simulink model "quaternion_simulation"  (R2022a)
settings: Solver=FixedStepAuto  StartTime=0.0  StopTime=60  FixedStep=Ts  RelTol=1e-3
values from neighbouring files (symbols this model uses):
  J_uav = diag([0.0118976 0.0118976 0.0218816])    [quaternion_simulation_init.m]
  K_att = [diag([100 100 3.16e-6]) diag([14.142 14.142 2.51e-3])]    [quaternion_simulation_init.m]
  K_pos = [diag([3.1622 3.1622 3.1622]) diag([2.7063 2.7063 2.7603])]    [quaternion_simulation_init.m]
  m_uav = 1.3    [quaternion_simulation_init.m]
  Ts = 0.005    [quaternion_simulation_init.m]
undefined symbols (not defined in the file or in its folder): sigbuilder_block
libraries: sharedtransform x2, SignalEditorBlockLib x1, uavutilslib x1
settings Model: PacingRate=3  Creator=marti  LastModifiedBy=martin
settings SolverCC: AlgebraicLoopSolver=TrustRegion
settings DebuggingCC: UnconnectedInputMsg=warning  UnconnectedOutputMsg=warning  UnconnectedLineMsg=warning  SFMachineParentedDataDiag=warning
settings RTWCC: DLArmComputeVersion=19.05

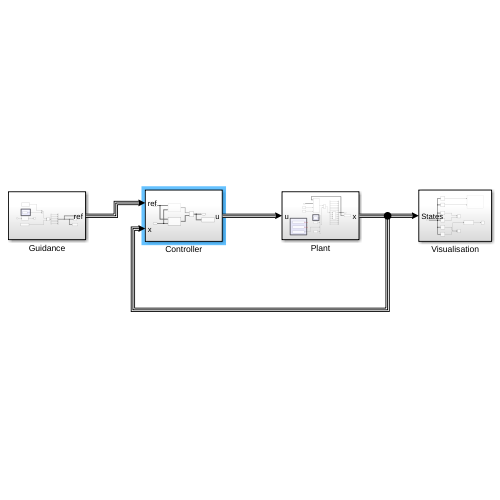
[thumbnail: Simulink's stored preview of the top-level diagram]
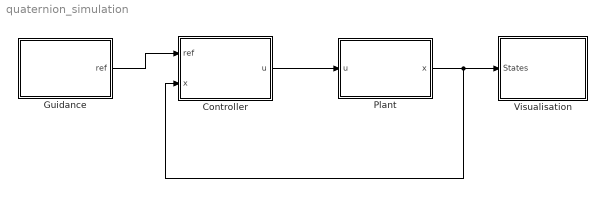
== system quaternion_simulation ==
  Controller : Subsystem
  Guidance : Subsystem
  Plant : Subsystem
  Visualisation : Subsystem
  wires:
  Guidance/1(ref) -> Controller/1(ref)
  Plant/1(x) -> Controller/2(x), Visualisation/1(States)
  Controller/1(u) -> Plant/1(u)

== system quaternion_simulation/Controller ==
  ref : Inport
  x : Inport  Port=2
  ADRC : Subsystem
  Manual Switch : ManualSwitch
  State-Feedback : Subsystem
  To Workspace : ToWorkspace  VariableName=control  SaveFormat=Timeseries  SampleTime=-1
  u : Outport
  wires:
  x/1 -> ADRC/2(x), State-Feedback/2(x)
  ref/1 -> State-Feedback/1(ref), ADRC/1(ref)
  ADRC/1(u) -> Manual Switch/2
  State-Feedback/1(u) -> Manual Switch/1
  Manual Switch/1 -> u/1, To Workspace/1

== system quaternion_simulation/Guidance ==
  note: velocity setpoints
  Bus Creator : BusCreator  Inputs=6
  Clock : Clock
  Constant : Constant  Value=[0;0;0]
  Demux : Demux  Outputs=6
  Fixed Setpoint : Constant  Value=[0; 0; 0; 0; 0; 0]
  Manual Switch : ManualSwitch  CurrentSetting=0
  Mux : Mux  Inputs=2
  Signal Editor : SignalEditorBlockLib/Signal Editor  FileName=/home/martin/thesis/ADRC_examples/Quaternion Simulation/trajectory.mat  ActiveScenario=square_1m_trajectory  ActiveSignal=Setpoint  IsBus=off  OutputBusObjectStr=Bus: BusObject  SampleTime=0  Interpolate=off  ZeroCross=off  OutputAfterFinalValue=Setting to zero  Unit=inherit  PreserveSignalName=on
  Terminator : Terminator
  To Workspace : ToWorkspace  VariableName=setpoints  SaveFormat=Timeseries  SampleTime=-1
  Trajectory : Scope
  Trajectory Generator : MATLAB Function  TreatAsAtomicUnit=on
  Out Bus Element : Outport  PortName=ref
  wires:
  Fixed Setpoint/1 -> Manual Switch/2
  Clock/1 -> Trajectory Generator/1(t)
  Constant/1 -> Mux/2
  Signal Editor/1 -> Mux/1
  Mux/1 -> Manual Switch/1
  Trajectory Generator/1(x_d) -> Terminator/1
  Manual Switch/1 -> Demux/1
  Demux/1 -> Bus Creator/1  "X"
  Demux/2 -> Bus Creator/2  "Y"
  Demux/3 -> Bus Creator/3  "Z"
  Demux/4 -> Bus Creator/4  "dX"
  Demux/5 -> Bus Creator/5  "dY"
  Demux/6 -> Bus Creator/6  "dZ"
  Bus Creator/1 -> Out Bus Element/1, To Workspace/1, Trajectory/1

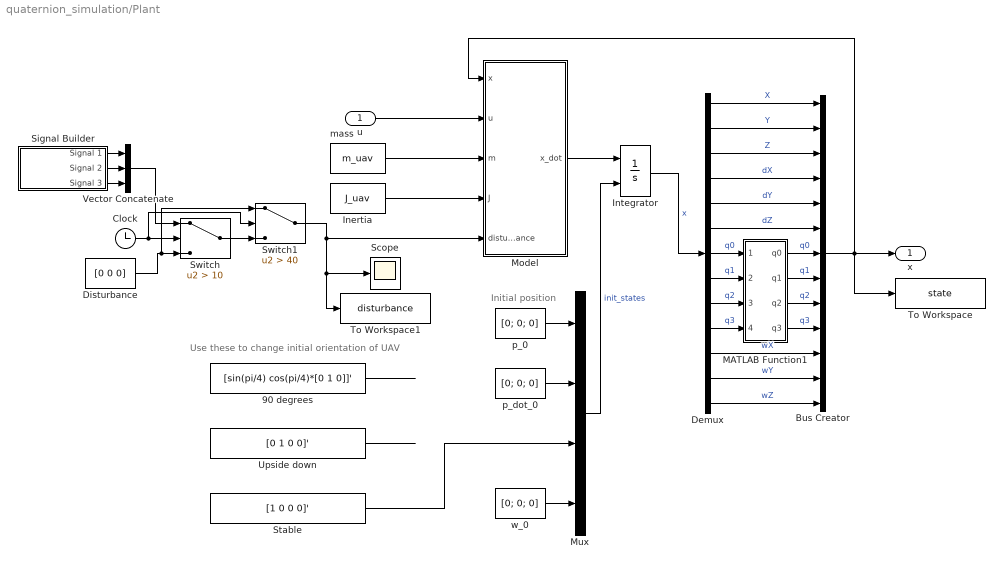
== system quaternion_simulation/Plant ==
  note: Initial position
  note: Use these to change initial orientation of UAV
  u : Inport
  90 degrees : Constant  Value=[sin(pi/4) cos(pi/4)*[0 1 0]]'  VectorParams1D=off
  Bus Creator : BusCreator  Inputs=13
  Clock : Clock
  Demux : Demux  Outputs=13
  Disturbance : Constant  Value=[0 0 0]  VectorParams1D=off
  Inertia : Constant  Value=J_uav  VectorParams1D=off
  Integrator : Integrator  InitialConditionSource=external
  MATLAB Function1 : MATLAB Function  TreatAsAtomicUnit=on
  Model : MATLAB Function  TreatAsAtomicUnit=on
  Mux : Mux
  Scope : Scope
  Signal Builder : Subsystem  Tag=STV Subsys  LoadFcn=sigbuilder_block('load');  StartFcn=sigbuilder_block('start');  StopFcn=sigbuilder_block('stop');  ClipboardFcn=sigbuilder_block('clipboard');  mask(Sigbuilder block){tuvar=[0:10]}
      mask help: Simulink:masks:SigbuilderBlock_MD
      mask init:
      | if ~strcmp(get_param(bdroot(gcbh),'SimulationStatus'),'stopped') tuvar = sigbuilder_block('maskInit'); end
      settings: CopyFcn=sigbuilder_block('copy');  DeleteFcn=sigbuilder_block('delete');  ModelCloseFcn=sigbuilder_block('modelClose');  PreSaveFcn=sigbuilder_block('preSave');  PauseFcn=sigbuilder_block('pause');  ContinueFcn=sigbuilder_block('continue');  NameChangeFcn=sigbuilder_block('namechange');  OpenFcn=sigbuilder_block('open',[437.6 3 550.4 399.75 ]);  CloseFcn=sigbuilder_block('close');
      mask Display: plot(0, 0, 100, 100,[2, 2, 32, 32, 2], [68, 8, 8, 68, 68],[32, 2], [38, 38], [32, 19, 2],[53, 60, 44], [32, 17, 17, 2],[16, 16, 31, 31]);txt = getActiveGroup(gcbh);text(2, 100, txt,'verticalAlignment', 'top');
  Stable : Constant  Value=[1 0 0 0]'  VectorParams1D=off
  Switch : Switch  Criteria=u2 > Threshold  Threshold=10  SaturateOnIntegerOverflow=off  InputSameDT=off
  Switch1 : Switch  Criteria=u2 > Threshold  Threshold=40  SaturateOnIntegerOverflow=off  InputSameDT=off
  To Workspace : ToWorkspace  VariableName=state  SaveFormat=Timeseries  SampleTime=-1
  To Workspace1 : ToWorkspace  VariableName=disturbance  SaveFormat=Timeseries  SampleTime=-1
  Upside down : Constant  Value=[0 1 0 0]'  VectorParams1D=off
  Vector Concatenate : Concatenate  NumInputs=3  Mode=Multidimensional array  ConcatenateDimension=2
  mass : Constant  Value=m_uav
  p_0 : Constant  Value=[0; 0; 0]  VectorParams1D=off
  p_dot_0 : Constant  Value=[0; 0; 0]  VectorParams1D=off
  w_0 : Constant  Value=[0; 0; 0]  VectorParams1D=off
  x : Outport
  wires:
  Inertia/1 -> Model/4(J)
  Model/1(x_dot) -> Integrator/1
  p_0/1 -> Mux/1
  p_dot_0/1 -> Mux/2
  w_0/1 -> Mux/4
  Integrator/1 -> Demux/1  "x"
  u/1 -> Model/2(u)
  Mux/1 -> Integrator/2  "init_states"
  Bus Creator/1 -> Model/1(x), To Workspace/1, x/1
  Demux/1 -> Bus Creator/1  "X"
  Demux/13 -> Bus Creator/13  "wZ"
  Demux/2 -> Bus Creator/2  "Y"
  Demux/3 -> Bus Creator/3  "Z"
  Demux/4 -> Bus Creator/4  "dX"
  Demux/5 -> Bus Creator/5  "dY"
  Demux/6 -> Bus Creator/6  "dZ"
  Demux/11 -> Bus Creator/11  "wX"
  Demux/12 -> Bus Creator/12  "wY"
  Demux/7 -> MATLAB Function1/1(q0_in)  "q0"
  Demux/8 -> MATLAB Function1/2(q1_in)  "q1"
  Demux/9 -> MATLAB Function1/3(q2_in)  "q2"
  Demux/10 -> MATLAB Function1/4(q3_in)  "q3"
  MATLAB Function1/1(q0) -> Bus Creator/7  "q0"
  MATLAB Function1/2(q1) -> Bus Creator/8  "q1"
  MATLAB Function1/3(q2) -> Bus Creator/9  "q2"
  MATLAB Function1/4(q3) -> Bus Creator/10  "q3"
  Stable/1 -> Mux/3
  mass/1 -> Model/3(m)
  90 degrees/1 -> ?
  Upside down/1 -> ?
  Vector Concatenate/1 -> Switch/1
  Clock/1 -> Switch1/2, Switch/2
  Disturbance/1 -> Switch1/1, Switch/3
  Signal Builder/1(Signal 1) -> Vector Concatenate/1
  Signal Builder/2(Signal 2) -> Vector Concatenate/2
  Signal Builder/3(Signal 3) -> Vector Concatenate/3
  Switch/1 -> Switch1/3
  Switch1/1 -> To Workspace1/1, Scope/1, Model/5(disturbance)

== system quaternion_simulation/Visualisation ==
  States : Inport
  Euler : Scope
  Linear : Scope  NumInputPorts=2
  Quaternion : Scope  NumInputPorts=2
  Quaternions to Rotation Angles : sharedtransform/Quaternions to Rotation Angles  rotationOrder=XYZ  aMode=aMode
      settings: SourceProductBaseCode=AE,PW,DR,MT,VE
  Selector : Selector  InputPortWidth=13  IndexOptions=Index vector (dialog)  Indices=[1:3]  OutputSizes=1
  Selector1 : Selector  InputPortWidth=13  IndexOptions=Index vector (dialog)  Indices=[4:6]  OutputSizes=1
  Selector2 : Selector  InputPortWidth=13  IndexOptions=Index vector (dialog)  Indices=[7:10]  OutputSizes=1
  Selector3 : Selector  InputPortWidth=13  IndexOptions=Index vector (dialog)  Indices=[11:13]  OutputSizes=1
  Selector4 : Selector  InputPortWidth=13  IndexOptions=Index vector (dialog)  Indices=[1:3]  OutputSizes=1
  Selector5 : Selector  InputPortWidth=13  IndexOptions=Index vector (dialog)  Indices=[7:10]  OutputSizes=1
  UAV Animation : uavutilslib/UAV Animation  Commented=on  UAVType=Multirotor  UAVSize=1  InertialZDirection=Up  SampleTime=-1
      settings: SourceProductBaseCode=UV
  wires:
  Selector2/1 -> Quaternions to Rotation Angles/1, Quaternion/1  "Orientation"
  States/1 -> Selector4/1, Selector5/1, Selector/1, Selector3/1, Selector2/1, Selector1/1
  Selector1/1 -> Linear/2  "Velocity"
  Selector/1 -> Linear/1  "Position"
  Selector3/1 -> Quaternion/2  "Angular Velocity"
  Selector5/1 -> UAV Animation/2  "Rotation"
  Selector4/1 -> UAV Animation/1  "Translation"
  Quaternions to Rotation Angles/1 -> Euler/1

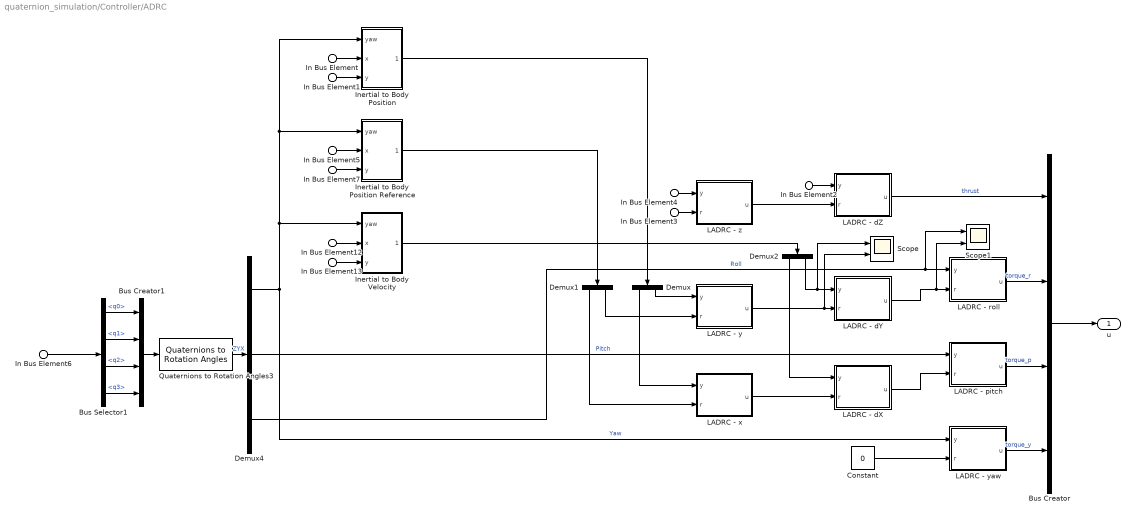
== system quaternion_simulation/Controller/ADRC ==
  In Bus Element7 : Inport  PortName=ref  Element=Y
  In Bus Element5 : Inport  PortName=ref  Element=X
  In Bus Element3 : Inport  PortName=ref  Element=Z
  In Bus Element6 : Inport  Port=2  PortName=x
  In Bus Element : Inport  Port=2  PortName=x  Element=X
  In Bus Element1 : Inport  Port=2  PortName=x  Element=Y
  In Bus Element12 : Inport  Port=2  PortName=x  Element=dX
  In Bus Element13 : Inport  Port=2  PortName=x  Element=dY
  In Bus Element4 : Inport  Port=2  PortName=x  Element=Z
  In Bus Element2 : Inport  Port=2  PortName=x  Element=dZ
  Bus Creator : BusCreator  Inputs=4
  Bus Creator1 : BusCreator  Inputs=4
  Bus Selector1 : BusSelector  OutputSignals=q0,q1,q2,q3
  Constant : Constant  Value=0
  Demux : Demux  Outputs=2
  Demux1 : Demux  Outputs=2
  Demux2 : Demux  Outputs=2
  Demux4 : Demux  Outputs=3
  Inertial to Body Position : Subsystem
  Inertial to Body Position Reference : Subsystem
  Inertial to Body Velocity : Subsystem
  LADRC - dX : Subsystem  VariantControl=Choice
  LADRC - dY : Subsystem  VariantControl=Choice
  LADRC - dZ : Subsystem  VariantControl=Choice
  LADRC - pitch : Subsystem  VariantControl=Choice
  LADRC - roll : Subsystem  VariantControl=Choice
  LADRC - x : Subsystem  VariantControl=Choice
  LADRC - y : Subsystem  VariantControl=Choice
  LADRC - yaw : Subsystem  VariantControl=Choice
  LADRC - z : Subsystem  VariantControl=Choice
  Quaternions to Rotation Angles3 : sharedtransform/Quaternions to Rotation Angles  rotationOrder=ZYX  aMode=aMode
      settings: SourceProductBaseCode=AE,PW,DR,MT,VE
  Scope : Scope  NumInputPorts=2
  Scope1 : Scope  NumInputPorts=2
  u : Outport
  wires:
  Bus Creator/1 -> u/1
  Demux4/3 -> Scope1/1, LADRC - roll/1(y)  "Roll"
  Bus Selector1/4 -> Bus Creator1/4  "<q3>"
  Bus Selector1/2 -> Bus Creator1/2  "<q1>"
  Bus Creator1/1 -> Quaternions to Rotation Angles3/1
  Bus Selector1/3 -> Bus Creator1/3  "<q2>"
  Bus Selector1/1 -> Bus Creator1/1  "<q0>"
  Demux4/1 -> LADRC - yaw/1(y), Inertial to Body Velocity/1(yaw), Inertial to Body Position/1(yaw), Inertial to Body Position Reference/1(yaw)  "Yaw"
  LADRC - dZ/1(u) -> Bus Creator/1  "thrust"
  Constant/1 -> LADRC - yaw/2(r)
  In Bus Element/1 -> Inertial to Body Position/2(x)
  In Bus Element1/1 -> Inertial to Body Position/3(y)
  In Bus Element13/1 -> Inertial to Body Velocity/3(y)
  LADRC - dY/1(u) -> Scope1/2, LADRC - roll/2(r)
  LADRC - dX/1(u) -> LADRC - pitch/2(r)
  In Bus Element6/1 -> Bus Selector1/1
  Quaternions to Rotation Angles3/1 -> Demux4/1  "ZYX"
  Demux4/2 -> LADRC - pitch/1(y)  "Pitch"
  Demux2/1 -> LADRC - dX/1(y)
  LADRC - yaw/1(u) -> Bus Creator/4  "torque_y"
  LADRC - pitch/1(u) -> Bus Creator/3  "torque_p"
  LADRC - roll/1(u) -> Bus Creator/2  "torque_r"
  In Bus Element3/1 -> LADRC - z/2(r)
  In Bus Element4/1 -> LADRC - z/1(y)
  In Bus Element5/1 -> Inertial to Body Position Reference/2(x)
  In Bus Element7/1 -> Inertial to Body Position Reference/3(y)
  In Bus Element12/1 -> Inertial to Body Velocity/2(x)
  LADRC - x/1(u) -> LADRC - dX/2(r)
  Inertial to Body Position/1(xy_body) -> Demux/1
  Demux/1 -> LADRC - x/1(y)
  Inertial to Body Position Reference/1(xy_body) -> Demux1/1
  Demux1/1 -> LADRC - x/2(r)
  Inertial to Body Velocity/1(xy_body) -> Demux2/1
  Demux2/2 -> Scope/1, LADRC - dY/1(y)
  LADRC - z/1(u) -> LADRC - dZ/2(r)
  LADRC - y/1(u) -> Scope/2, LADRC - dY/2(r)
  Demux1/2 -> LADRC - y/2(r)
  In Bus Element2/1 -> LADRC - dZ/1(y)
  Demux/2 -> LADRC - y/1(y)

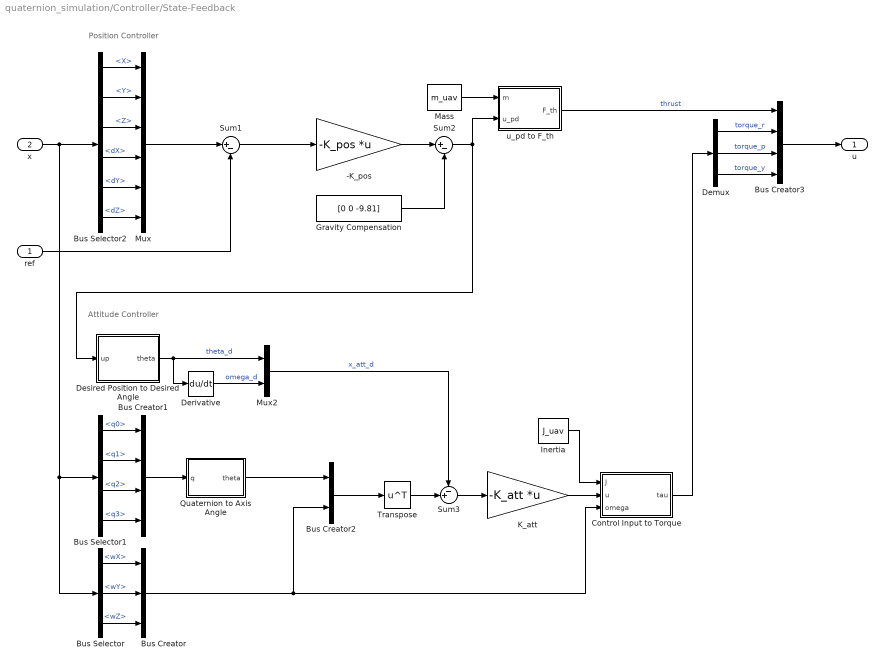
== system quaternion_simulation/Controller/State-Feedback ==
  note: Attitude Controller
  note: Position Controller
  ref : Inport
  x : Inport  Port=2
  -K_pos : Gain  Gain=-K_pos  Multiplication=Matrix(K*u) (u vector)
  Bus Creator : BusCreator  Inputs=3
  Bus Creator1 : BusCreator  Inputs=4
  Bus Creator2 : BusCreator  Inputs=2
  Bus Creator3 : BusCreator  Inputs=4
  Bus Selector : BusSelector  OutputSignals=wX,wY,wZ
  Bus Selector1 : BusSelector  OutputSignals=q0,q1,q2,q3
  Bus Selector2 : BusSelector  OutputSignals=X,Y,Z,dX,dY,dZ
  Control Input to Torque : MATLAB Function  TreatAsAtomicUnit=on
  Demux : Demux  Outputs=3
  Derivative : Derivative
  Desired Position to Desired Angle : MATLAB Function  TreatAsAtomicUnit=on
  Gravity Compensation : Constant  Value=[0 0 -9.81]
  Inertia : Constant  Value=J_uav  VectorParams1D=off
  K_att : Gain  Gain=-K_att  Multiplication=Matrix(K*u) (u vector)
  Mass : Constant  Value=m_uav
  Mux : Mux  Inputs=6
  Mux2 : Mux  Inputs=2
  Quaternion to Axis Angle : MATLAB Function  TreatAsAtomicUnit=on
  Sum1 : Sum  Inputs=|+-
  Sum2 : Sum  Inputs=|+-
  Sum3 : Sum  Inputs=-+|
  Transpose : Math  Operator=transpose
  u_pd to F_th : MATLAB Function  TreatAsAtomicUnit=on
  u : Outport
  wires:
  u_pd to F_th/1(F_th) -> Bus Creator3/1  "thrust"
  Bus Selector1/1 -> Bus Creator1/1  "<q0>"
  x/1 -> Bus Selector/1, Bus Selector1/1, Bus Selector2/1
  Bus Selector1/3 -> Bus Creator1/3  "<q2>"
  Bus Selector2/3 -> Mux/3  "<Z>"
  Bus Selector/3 -> Bus Creator/3  "<wZ>"
  Bus Selector2/1 -> Mux/1  "<X>"
  Bus Creator/1 -> Bus Creator2/2, Control Input to Torque/3(omega)
  Bus Selector2/6 -> Mux/6  "<dZ>"
  Bus Selector2/5 -> Mux/5  "<dY>"
  Bus Selector2/4 -> Mux/4  "<dX>"
  Bus Selector1/4 -> Bus Creator1/4  "<q3>"
  Bus Selector2/2 -> Mux/2  "<Y>"
  Bus Creator2/1 -> Transpose/1
  Bus Selector1/2 -> Bus Creator1/2  "<q1>"
  Quaternion to Axis Angle/1(theta) -> Bus Creator2/1
  Bus Selector/2 -> Bus Creator/2  "<wY>"
  Bus Selector/1 -> Bus Creator/1  "<wX>"
  Mass/1 -> u_pd to F_th/1(m)
  ref/1 -> Sum1/2
  Gravity Compensation/1 -> Sum2/2
  Sum2/1 -> u_pd to F_th/2(u_pd), Desired Position to Desired Angle/1(up)
  Sum1/1 -> -K_pos/1
  Mux/1 -> Sum1/1
  Inertia/1 -> Control Input to Torque/1(J)
  Bus Creator1/1 -> Quaternion to Axis Angle/1(q)
  -K_pos/1 -> Sum2/1
  Sum3/1 -> K_att/1
  K_att/1 -> Control Input to Torque/2(u)
  Control Input to Torque/1(tau) -> Demux/1
  Derivative/1 -> Mux2/2  "omega_d"
  Desired Position to Desired Angle/1(theta) -> Derivative/1, Mux2/1  "theta_d"
  Transpose/1 -> Sum3/2
  Mux2/1 -> Sum3/1  "x_att_d"
  Bus Creator3/1 -> u/1
  Demux/2 -> Bus Creator3/3  "torque_p"
  Demux/1 -> Bus Creator3/2  "torque_r"
  Demux/3 -> Bus Creator3/4  "torque_y"

== system quaternion_simulation/Plant/Signal Builder ==
  Demux : Demux  Tag=STV Demux  Outputs=3
      settings: DisplayOption=none
  FromWs : FromWorkspace  Tag=STV FromWs  VariableName=tuvar
      SigBuilderData=|
      | common.afterFinalStr = 'Extrapolate'
      | common.sampleTime = 0
      | dataSet.timeRange = [0 100]
      | dataSet.name = 'Group 1'
      | sbobj.Groups.Name = 'Group 1'
      | sbobj.Groups.Signals(1).Name = 'Signal 1'
      | sbobj.Groups.Signals(1).XData = [0 2 4 6 8 10 12 14 16 18 20 22 24 26 28 30 32 34 36 38 40 42 44 46 48 50 52 54 56 58 60 62 64 66 68 70 72 74 76 78 80 82 84 86 88 90 92 94 96 98 100]
      | sbobj.Groups.Signals(1).YData = [0.949221831131 0.307061919147 0.135174942099 0.515246335525 0.261406324055 -0.941485770955 -0.162337672804 -0.146054634332 -0.532011376809 1.68210359466 -0.87572934616 -0.48381505011 -0.712004549027 -1.17421233146 -0.192239517539 -0.274070229933 1.53007251442 -0.249024742514 -1.06421341289 1.60345729812 1.23467914689 -0.229626450963 -1.50615970398 -0.444627816447 -0.155941035725 0.276068253932 -0.261163645776 0.443421912904 0.391894209432 -1.25067890683 -0.947960922331 -0.74110609394 -0.507817550278 -0.3205755066 0.0124690413616 -3.0291773414 -0.457014640872 1.24244840639 -1.06670139898 0.933728162671 0.350321001356 -0.0290057637087 0.182452167506 -1.56505601415 -0.0845394798177 1.6039463506 0.0983477746401 0.0413736134896 -0.734169112697 -0.0308137300123 0.232347012624]
      | sbobj.Groups.Signals(2).Name = 'Signal 2'
      | sbobj.Groups.Signals(2).XData = [0 1 2 3 4 5 6 7 8 9 10 11 12 13 14 15 16 17 18 19 20 21 22 23 24 25 26 27 28 29 30 31 32 33 34 35 36 37 38 39 40 41 42 43 44 45 46 47 48 49 50 51 52 53 54 55 56 57 58 59 60 61 62 63 64 65 66 67 68 69 70 71 72 73 74 75 76 77 78 79 80 81 82 83 84 85 86 87 88 89 90 91 92 93 94 95 96 97 98 99 100]
      | sbobj.Groups.Signals(2).YData = [-0.888032082329 0.100092833139 -0.544528929991 0.303520794649 -0.600326562134 0.489965321174 0.739363123604 1.71188778298 -0.194123535758 -2.13835526944 -0.839588747337 1.354594328 -1.07215528838 0.960953869741 0.124049800003 1.43669662272 -1.96089999937 -0.197698225974 -1.20784548526 2.90800803073 0.825218894228 1.37897197792 -1.05818025799 -0.468615581101 -0.27246940925 1.09842461789 -0.277871932788 0.701541458163 -2.05181629991 -0.353849997774 -0.823586525157 -1.5770570228 0.507974650906 0.281984063671 0.0334798822445 -1.33367794343 1.12749227834 0.350179410603 -0.299066030333 0.0228897927516 -0.261995434966 -1.75021236845 -0.285650971595 -0.831366511568 -0.979206305167 -1.15640165566 -0.533557109316 -2.00263573588 0.964229422632 0.520060101455 -0.0200278516425 -0.0347710860285 -0.798163584564 1.01868528213 -0.133217479508 -0.714530163787 1.35138576843 -0.224771056053 -0.589029030721 -0.293753597735 -0.847926243638 -1.12012830124 2.52599969212 1.65549759289 0.307535159238 -1.25711835935 -0.865468030555 -0.176534114231 0.791416061629 -1.33200442132 -2.32986715581 -1.44909729284 0.333510833066 0.391353604433 0.451679418928 -0.130284653146 0.183689095862 -0.476153016619 0.862021611557 -1.36169447087 0.455029556444 -0.848709379934 -0.334886938964 0.552783345945 1.0390906535 -1.11763868327 1.26065870912 0.660143141047 -0.0678655535427 -0.195221197899 -0.217606350143 -0.303107621352 0.0230456244251 0.0512903558488 0.826062790212 1.52697668673 0.466914435685 -0.209713338389 0.625190357088 0.183227263001 -1.02976754357]
      | sbobj.Groups.Signals(3).Name = 'Signal 3'
      | sbobj.Groups.Signals(3).XData = [0 1 2 3 4 5 6 7 8 9 10 11 12 13 14 15 16 17 18 19 20 21 22 23 24 25 26 27 28 29 30 31 32 33 34 35 36 37 38 39 40 41 42 43 44 45 46 47 48 49 50 51 52 53 54 55 56 57 58 59 60 61 62 63 64 65 66 67 68 69 70 71 72 73 74 75 76 77 78 79 80 81 82 83 84 85 86 87 88 89 90 91 92 93 94 95 96 97 98 99 100]
      | sbobj.Groups.Signals(3).YData = [0.537667139546 1.8338850146 -2.258846861 0.862173320368 0.318765239859 -1.30768829631 -0.433592022306 0.342624466539 3.57839693973 2.76943702988 -1.34988694016 3.03492346633 0.725404224946 -0.0630548731897 0.714742903826 -0.2049660583 -0.124144348216 1.48969760779 1.4090344898 1.41719241343 0.671497133608 -1.20748692269 0.717238651329 1.63023528916 0.488893770312 1.03469300992 0.726885133383 -0.303440924786 0.293871467097 -0.787282803759 0.888395631758 -1.14707010697 -1.06887045817 -0.809498694425 -2.94428416199 1.43838029282 0.325190539456 -0.75492831917 1.3702985401 -1.71151641885 -0.102242446085 -0.241447041607 0.319206739166 0.312858596637 -0.864879917324 -0.0300512961963 -0.164879019209 0.627707287529 1.09326566904 1.10927329761 -0.863652821989 0.0773590911304 -1.21411704362 -1.11350074149 -0.00684932810335 1.53263030828 -0.769665913754 0.37137881276 -0.225584402271 1.11735613881 -1.08906429505 0.032557464165 0.552527021112 1.10061021788 1.5442118955 0.0859311331754 -1.49159031064 -0.74230183726 -1.06158173332 2.350457224 -0.615601881467 0.748076783704 -0.192418510588 0.888610425421 -0.764849236568 -1.40226896934 -1.42237592509 0.48819390986 -0.177375156619 -0.196053487807 1.41931015064 0.291584373984 0.197811053464 1.58769908997 -0.80446595635 0.69662441585 0.835088165073 -0.243715140378 0.215670086404 -1.16584393148 -1.1479527789 0.104874716016 0.722254032225 2.58549125262 -0.666890670701 0.187331024579 -0.082494425371 -1.93302291785 -0.438966153935 -1.79467884146 0.840375529754]
      | sbobj.Groups.TimeRange = [0 100]
  Signal 1 : Outport  Tag=STV Outport
  Signal 2 : Outport  Tag=STV Outport  Port=2
  Signal 3 : Outport  Tag=STV Outport  Port=3
  wires:
  Demux/1 -> Signal 1/1
  FromWs/1 -> Demux/1
  Demux/2 -> Signal 2/1
  Demux/3 -> Signal 3/1

== system quaternion_simulation/Controller/ADRC/Inertial to Body Position ==
  yaw : Inport
  x : Inport  Port=2
  y : Inport  Port=3
  Gain : Gain  Gain=-1
  Matrix Concatenate : Concatenate  Mode=Multidimensional array  ConcatenateDimension=2
  MatrixMultiply : Product  Multiplication=Matrix(*)
  Trigonometric Function : Trigonometry  Operator=sincos
  Vector Concatenate : Concatenate
  Vector Concatenate1 : Concatenate
  Vector Concatenate2 : Concatenate
  xy_body : Outport
  wires:
  Trigonometric Function/2 -> Vector Concatenate1/2, Vector Concatenate/1
  Trigonometric Function/1 -> Vector Concatenate1/1, Gain/1
  Gain/1 -> Vector Concatenate/2
  Matrix Concatenate/1 -> MatrixMultiply/1
  MatrixMultiply/1 -> xy_body/1
  Vector Concatenate2/1 -> MatrixMultiply/2
  Vector Concatenate/1 -> Matrix Concatenate/1
  Vector Concatenate1/1 -> Matrix Concatenate/2
  y/1 -> Vector Concatenate2/2
  x/1 -> Vector Concatenate2/1
  yaw/1 -> Trigonometric Function/1

== system quaternion_simulation/Controller/ADRC/Inertial to Body Position Reference ==
  yaw : Inport
  x : Inport  Port=2
  y : Inport  Port=3
  Gain : Gain  Gain=-1
  Matrix Concatenate : Concatenate  Mode=Multidimensional array  ConcatenateDimension=2
  MatrixMultiply : Product  Multiplication=Matrix(*)
  Trigonometric Function : Trigonometry  Operator=sincos
  Vector Concatenate : Concatenate
  Vector Concatenate1 : Concatenate
  Vector Concatenate2 : Concatenate
  xy_body : Outport
  wires:
  Trigonometric Function/2 -> Vector Concatenate1/2, Vector Concatenate/1
  Trigonometric Function/1 -> Vector Concatenate1/1, Gain/1
  Gain/1 -> Vector Concatenate/2
  Matrix Concatenate/1 -> MatrixMultiply/1
  MatrixMultiply/1 -> xy_body/1
  Vector Concatenate2/1 -> MatrixMultiply/2
  Vector Concatenate/1 -> Matrix Concatenate/1
  Vector Concatenate1/1 -> Matrix Concatenate/2
  y/1 -> Vector Concatenate2/2
  x/1 -> Vector Concatenate2/1
  yaw/1 -> Trigonometric Function/1

== system quaternion_simulation/Controller/ADRC/Inertial to Body Velocity ==
  yaw : Inport
  x : Inport  Port=2
  y : Inport  Port=3
  Gain : Gain  Gain=-1
  Matrix Concatenate : Concatenate  Mode=Multidimensional array  ConcatenateDimension=2
  MatrixMultiply : Product  Multiplication=Matrix(*)
  Trigonometric Function : Trigonometry  Operator=sincos
  Vector Concatenate : Concatenate
  Vector Concatenate1 : Concatenate
  Vector Concatenate2 : Concatenate
  xy_body : Outport
  wires:
  Trigonometric Function/2 -> Vector Concatenate1/2, Vector Concatenate/1
  Trigonometric Function/1 -> Vector Concatenate1/1, Gain/1
  Gain/1 -> Vector Concatenate/2
  Matrix Concatenate/1 -> MatrixMultiply/1
  MatrixMultiply/1 -> xy_body/1
  Vector Concatenate2/1 -> MatrixMultiply/2
  Vector Concatenate/1 -> Matrix Concatenate/1
  Vector Concatenate1/1 -> Matrix Concatenate/2
  y/1 -> Vector Concatenate2/2
  x/1 -> Vector Concatenate2/1
  yaw/1 -> Trigonometric Function/1

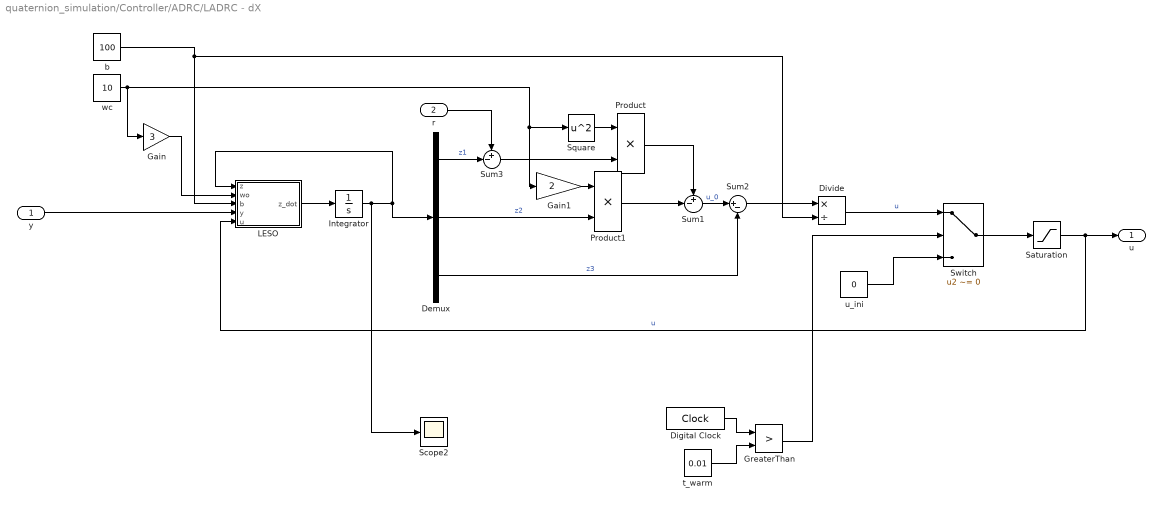
== system quaternion_simulation/Controller/ADRC/LADRC - dX ==
  y : Inport
  r : Inport  Port=2
  Demux : Demux  Outputs=3
  Digital Clock : DigitalClock  SampleTime=Ts
  Divide : Product  Inputs=*/
  Gain : Gain  Gain=3
  Gain1 : Gain  Gain=2
  GreaterThan : RelationalOperator  Operator=>  OutDataTypeStr=boolean  RndMeth=Simplest  InputSameDT=off
  Integrator : Integrator  InitialCondition=[0 0 0]'
  LESO : MATLAB Function  TreatAsAtomicUnit=on
  Product : Product
  Product1 : Product
  Saturation : Saturate  UpperLimit=pi/8  LowerLimit=-pi/8
  Scope2 : Scope
  Square : Math  Operator=square
  Sum1 : Sum  Inputs=+-|
  Sum2 : Sum  Inputs=|+-
  Sum3 : Sum  Inputs=+-|
  Switch : Switch  Criteria=u2 ~= 0  Threshold=0.1  SaturateOnIntegerOverflow=off  InputSameDT=off
  b : Constant  Value=100
  t_warm : Constant  Value=0.01
  u_ini : Constant  Value=0  OutDataTypeStr=single
  wc : Constant  Value=10
  u : Outport
  wires:
  LESO/1(z_dot) -> Integrator/1
  Integrator/1 -> Scope2/1, LESO/1(z), Demux/1
  Demux/1 -> Sum3/2  "z1"
  Product/1 -> Sum1/1
  Sum1/1 -> Sum2/1  "u_0"
  Demux/3 -> Sum2/2  "z3"
  Sum2/1 -> Divide/1
  Square/1 -> Product/1
  Gain1/1 -> Product1/1
  Demux/2 -> Product1/2  "z2"
  Product1/1 -> Sum1/2
  Saturation/1 -> LESO/5(u), u/1  "u"
  Switch/1 -> Saturation/1
  Divide/1 -> Switch/1  "u"
  u_ini/1 -> Switch/3
  r/1 -> Sum3/1
  Sum3/1 -> Product/2
  b/1 -> Divide/2, LESO/3(b)
  wc/1 -> Gain/1, Gain1/1, Square/1
  Gain/1 -> LESO/2(wo)
  t_warm/1 -> GreaterThan/2
  Digital Clock/1 -> GreaterThan/1
  GreaterThan/1 -> Switch/2
  y/1 -> LESO/4(y)

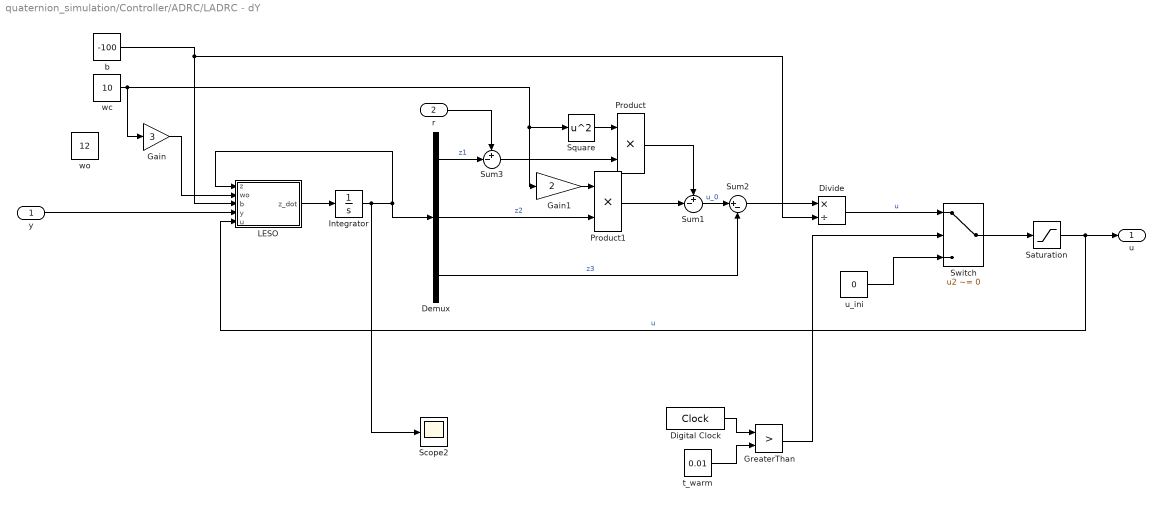
== system quaternion_simulation/Controller/ADRC/LADRC - dY ==
  y : Inport
  r : Inport  Port=2
  Demux : Demux  Outputs=3
  Digital Clock : DigitalClock  SampleTime=Ts
  Divide : Product  Inputs=*/
  Gain : Gain  Gain=3
  Gain1 : Gain  Gain=2
  GreaterThan : RelationalOperator  Operator=>  OutDataTypeStr=boolean  RndMeth=Simplest  InputSameDT=off
  Integrator : Integrator  InitialCondition=[0 0 0]'
  LESO : MATLAB Function  TreatAsAtomicUnit=on
  Product : Product
  Product1 : Product
  Saturation : Saturate  UpperLimit=pi/8  LowerLimit=-pi/8
  Scope2 : Scope
  Square : Math  Operator=square
  Sum1 : Sum  Inputs=+-|
  Sum2 : Sum  Inputs=|+-
  Sum3 : Sum  Inputs=+-|
  Switch : Switch  Criteria=u2 ~= 0  Threshold=0.1  SaturateOnIntegerOverflow=off  InputSameDT=off
  b : Constant  Value=-100
  t_warm : Constant  Value=0.01
  u_ini : Constant  Value=0  OutDataTypeStr=single
  wc : Constant  Value=10
  wo : Constant  Value=12
  u : Outport
  wires:
  LESO/1(z_dot) -> Integrator/1
  Integrator/1 -> Scope2/1, LESO/1(z), Demux/1
  Demux/1 -> Sum3/2  "z1"
  Product/1 -> Sum1/1
  Sum1/1 -> Sum2/1  "u_0"
  Demux/3 -> Sum2/2  "z3"
  Sum2/1 -> Divide/1
  Square/1 -> Product/1
  Gain1/1 -> Product1/1
  Demux/2 -> Product1/2  "z2"
  Product1/1 -> Sum1/2
  Saturation/1 -> LESO/5(u), u/1  "u"
  Switch/1 -> Saturation/1
  Divide/1 -> Switch/1  "u"
  u_ini/1 -> Switch/3
  r/1 -> Sum3/1
  Sum3/1 -> Product/2
  b/1 -> Divide/2, LESO/3(b)
  wc/1 -> Gain/1, Gain1/1, Square/1
  Gain/1 -> LESO/2(wo)
  t_warm/1 -> GreaterThan/2
  Digital Clock/1 -> GreaterThan/1
  GreaterThan/1 -> Switch/2
  y/1 -> LESO/4(y)

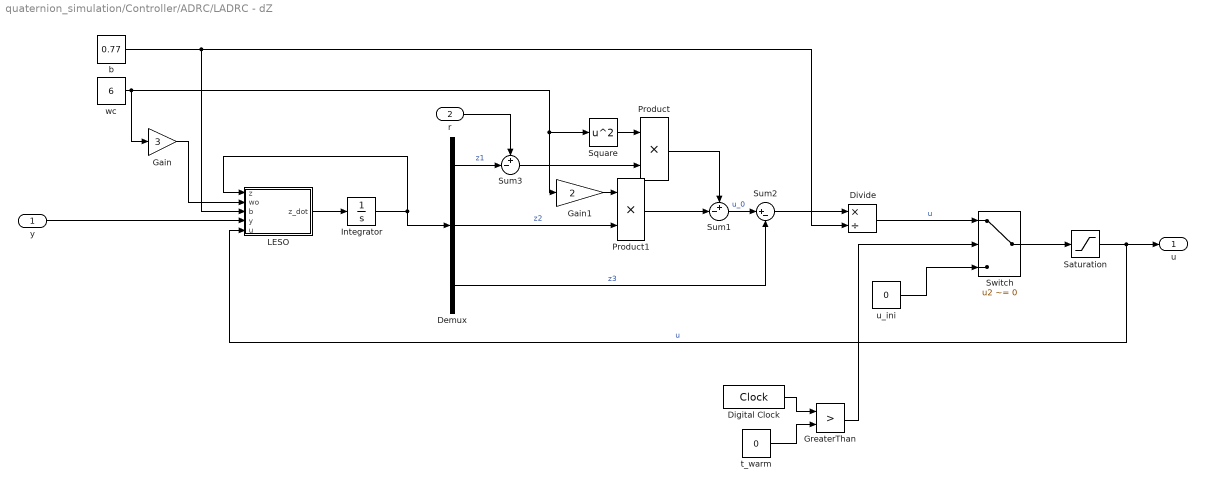
== system quaternion_simulation/Controller/ADRC/LADRC - dZ ==
  y : Inport
  r : Inport  Port=2
  Demux : Demux  Outputs=3
  Digital Clock : DigitalClock  SampleTime=Ts
  Divide : Product  Inputs=*/
  Gain : Gain  Gain=3
  Gain1 : Gain  Gain=2
  GreaterThan : RelationalOperator  Operator=>  OutDataTypeStr=boolean  RndMeth=Simplest  InputSameDT=off
  Integrator : Integrator  InitialCondition=[0 0 -9.81]'
  LESO : MATLAB Function  TreatAsAtomicUnit=on
  Product : Product
  Product1 : Product
  Saturation : Saturate  UpperLimit=30  LowerLimit=0
  Square : Math  Operator=square
  Sum1 : Sum  Inputs=+-|
  Sum2 : Sum  Inputs=|+-
  Sum3 : Sum  Inputs=+-|
  Switch : Switch  Criteria=u2 ~= 0  Threshold=0.1  SaturateOnIntegerOverflow=off  InputSameDT=off
  b : Constant  Value=0.77
  t_warm : Constant  Value=0
  u_ini : Constant  Value=0  OutDataTypeStr=single
  wc : Constant  Value=6
  u : Outport
  wires:
  LESO/1(z_dot) -> Integrator/1
  Integrator/1 -> LESO/1(z), Demux/1
  Demux/1 -> Sum3/2  "z1"
  Product/1 -> Sum1/1
  Sum1/1 -> Sum2/1  "u_0"
  Demux/3 -> Sum2/2  "z3"
  Sum2/1 -> Divide/1
  Square/1 -> Product/1
  Gain1/1 -> Product1/1
  Demux/2 -> Product1/2  "z2"
  Product1/1 -> Sum1/2
  Saturation/1 -> LESO/5(u), u/1  "u"
  Switch/1 -> Saturation/1
  Divide/1 -> Switch/1  "u"
  u_ini/1 -> Switch/3
  r/1 -> Sum3/1
  Sum3/1 -> Product/2
  b/1 -> LESO/3(b), Divide/2
  wc/1 -> Gain/1, Gain1/1, Square/1
  Gain/1 -> LESO/2(wo)
  t_warm/1 -> GreaterThan/2
  Digital Clock/1 -> GreaterThan/1
  GreaterThan/1 -> Switch/2
  y/1 -> LESO/4(y)

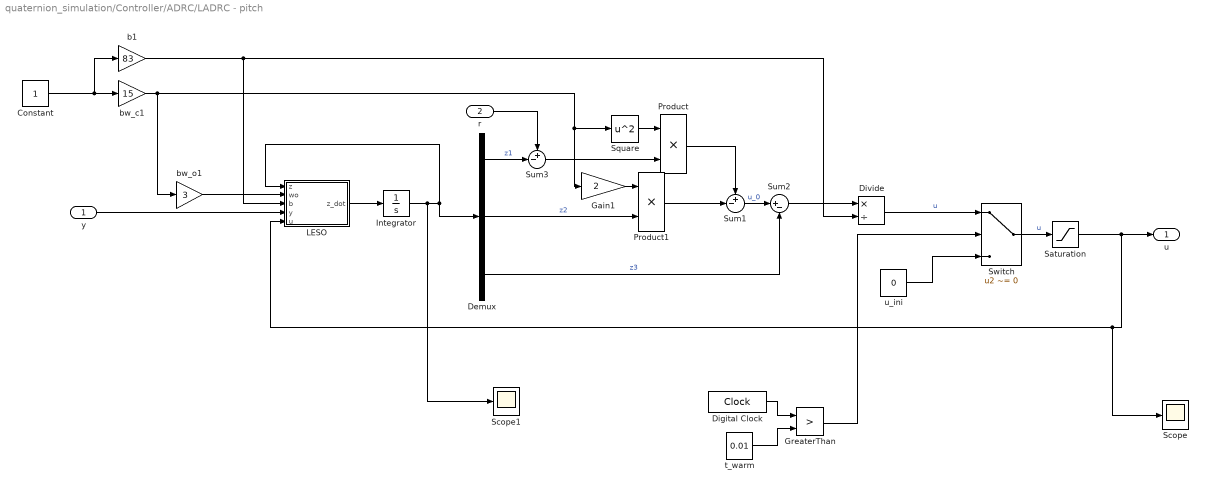
== system quaternion_simulation/Controller/ADRC/LADRC - pitch ==
  y : Inport
  r : Inport  Port=2
  Constant : Constant
  Demux : Demux  Outputs=3
  Digital Clock : DigitalClock  SampleTime=Ts
  Divide : Product  Inputs=*/
  Gain1 : Gain  Gain=2
  GreaterThan : RelationalOperator  Operator=>  OutDataTypeStr=boolean  RndMeth=Simplest  InputSameDT=off
  Integrator : Integrator  InitialCondition=[0 0 0]'
  LESO : MATLAB Function  TreatAsAtomicUnit=on
  Product : Product
  Product1 : Product
  Saturation : Saturate  UpperLimit=0.25  LowerLimit=-0.25
  Scope : Scope
  Scope1 : Scope
  Square : Math  Operator=square
  Sum1 : Sum  Inputs=+-|
  Sum2 : Sum  Inputs=|+-
  Sum3 : Sum  Inputs=+-|
  Switch : Switch  Criteria=u2 ~= 0  Threshold=0.1  SaturateOnIntegerOverflow=off  InputSameDT=off
  b1 : Gain  Gain=83
  bw_c1 : Gain  Gain=15
  bw_o1 : Gain  Gain=3
  t_warm : Constant  Value=0.01
  u_ini : Constant  Value=0  OutDataTypeStr=single
  u : Outport
  wires:
  LESO/1(z_dot) -> Integrator/1
  Integrator/1 -> Scope1/1, LESO/1(z), Demux/1
  Demux/1 -> Sum3/2  "z1"
  Product/1 -> Sum1/1
  Sum1/1 -> Sum2/1  "u_0"
  Demux/3 -> Sum2/2  "z3"
  Sum2/1 -> Divide/1
  Square/1 -> Product/1
  Gain1/1 -> Product1/1
  Demux/2 -> Product1/2  "z2"
  Product1/1 -> Sum1/2
  Switch/1 -> Saturation/1  "u"
  Divide/1 -> Switch/1  "u"
  u_ini/1 -> Switch/3
  r/1 -> Sum3/1
  Sum3/1 -> Product/2
  b1/1 -> Divide/2, LESO/3(b)
  bw_c1/1 -> bw_o1/1, Gain1/1, Square/1
  bw_o1/1 -> LESO/2(wo)
  t_warm/1 -> GreaterThan/2
  Digital Clock/1 -> GreaterThan/1
  GreaterThan/1 -> Switch/2
  y/1 -> LESO/4(y)
  Constant/1 -> bw_c1/1, b1/1
  Saturation/1 -> Scope/1, LESO/5(u), u/1

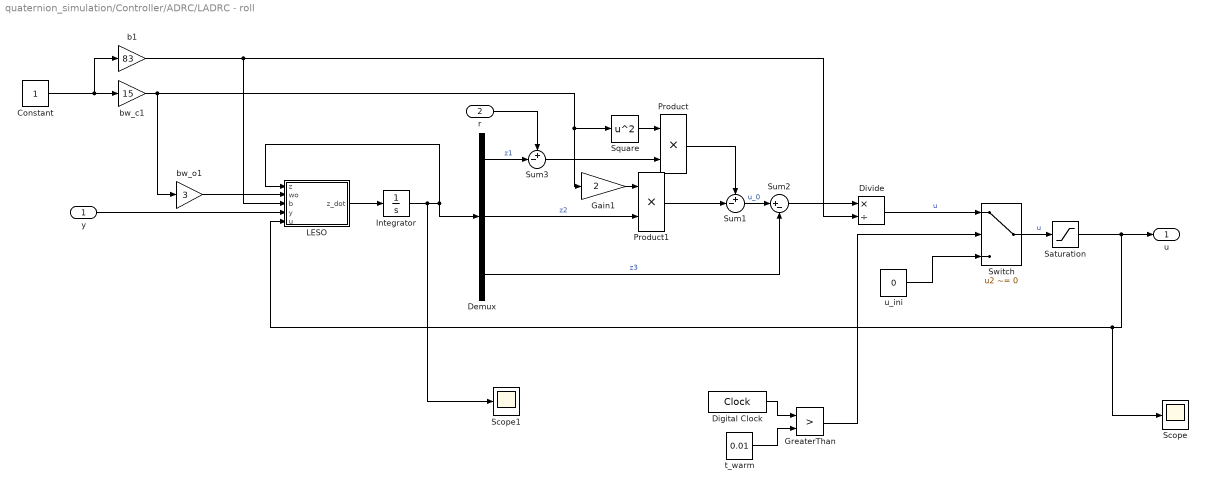
== system quaternion_simulation/Controller/ADRC/LADRC - roll ==
  y : Inport
  r : Inport  Port=2
  Constant : Constant
  Demux : Demux  Outputs=3
  Digital Clock : DigitalClock  SampleTime=Ts
  Divide : Product  Inputs=*/
  Gain1 : Gain  Gain=2
  GreaterThan : RelationalOperator  Operator=>  OutDataTypeStr=boolean  RndMeth=Simplest  InputSameDT=off
  Integrator : Integrator  InitialCondition=[0 0 0]'
  LESO : MATLAB Function  TreatAsAtomicUnit=on
  Product : Product
  Product1 : Product
  Saturation : Saturate  UpperLimit=0.25  LowerLimit=-0.25
  Scope : Scope
  Scope1 : Scope
  Square : Math  Operator=square
  Sum1 : Sum  Inputs=+-|
  Sum2 : Sum  Inputs=|+-
  Sum3 : Sum  Inputs=+-|
  Switch : Switch  Criteria=u2 ~= 0  Threshold=0.1  SaturateOnIntegerOverflow=off  InputSameDT=off
  b1 : Gain  Gain=83
  bw_c1 : Gain  Gain=15
  bw_o1 : Gain  Gain=3
  t_warm : Constant  Value=0.01
  u_ini : Constant  Value=0  OutDataTypeStr=single
  u : Outport
  wires:
  LESO/1(z_dot) -> Integrator/1
  Integrator/1 -> Scope1/1, LESO/1(z), Demux/1
  Demux/1 -> Sum3/2  "z1"
  Product/1 -> Sum1/1
  Sum1/1 -> Sum2/1  "u_0"
  Demux/3 -> Sum2/2  "z3"
  Sum2/1 -> Divide/1
  Square/1 -> Product/1
  Gain1/1 -> Product1/1
  Demux/2 -> Product1/2  "z2"
  Product1/1 -> Sum1/2
  Switch/1 -> Saturation/1  "u"
  Divide/1 -> Switch/1  "u"
  u_ini/1 -> Switch/3
  r/1 -> Sum3/1
  Sum3/1 -> Product/2
  b1/1 -> Divide/2, LESO/3(b)
  bw_c1/1 -> bw_o1/1, Gain1/1, Square/1
  bw_o1/1 -> LESO/2(wo)
  t_warm/1 -> GreaterThan/2
  Digital Clock/1 -> GreaterThan/1
  GreaterThan/1 -> Switch/2
  y/1 -> LESO/4(y)
  Constant/1 -> bw_c1/1, b1/1
  Saturation/1 -> Scope/1, LESO/5(u), u/1

== system quaternion_simulation/Controller/ADRC/LADRC - x ==
  y : Inport
  r : Inport  Port=2
  Demux : Demux  Outputs=3
  Digital Clock : DigitalClock  SampleTime=Ts
  Divide : Product  Inputs=*/
  Gain : Gain  Gain=3
  Gain1 : Gain  Gain=2
  GreaterThan : RelationalOperator  Operator=>  OutDataTypeStr=boolean  RndMeth=Simplest  InputSameDT=off
  Integrator : Integrator  InitialCondition=[0 0 0]'
  LESO : MATLAB Function  TreatAsAtomicUnit=on
  Product : Product
  Product1 : Product
  Saturation : Saturate  UpperLimit=3  LowerLimit=-3
  Square : Math  Operator=square
  Sum1 : Sum  Inputs=+-|
  Sum2 : Sum  Inputs=|+-
  Sum3 : Sum  Inputs=+-|
  Switch : Switch  Criteria=u2 ~= 0  Threshold=0.1  SaturateOnIntegerOverflow=off  InputSameDT=off
  b : Constant  Value=10
  t_warm : Constant  Value=0.01
  u_ini : Constant  Value=0  OutDataTypeStr=single
  wc : Constant  Value=3
  u : Outport
  wires:
  LESO/1(z_dot) -> Integrator/1
  Integrator/1 -> LESO/1(z), Demux/1
  Demux/1 -> Sum3/2  "z1"
  Product/1 -> Sum1/1
  Sum1/1 -> Sum2/1  "u_0"
  Demux/3 -> Sum2/2  "z3"
  Sum2/1 -> Divide/1
  Square/1 -> Product/1
  Gain1/1 -> Product1/1
  Demux/2 -> Product1/2  "z2"
  Product1/1 -> Sum1/2
  Saturation/1 -> LESO/5(u), u/1  "u"
  Switch/1 -> Saturation/1
  Divide/1 -> Switch/1  "u"
  u_ini/1 -> Switch/3
  r/1 -> Sum3/1
  Sum3/1 -> Product/2
  b/1 -> Divide/2, LESO/3(b)
  wc/1 -> Gain/1, Gain1/1, Square/1
  Gain/1 -> LESO/2(wo)
  t_warm/1 -> GreaterThan/2
  Digital Clock/1 -> GreaterThan/1
  GreaterThan/1 -> Switch/2
  y/1 -> LESO/4(y)

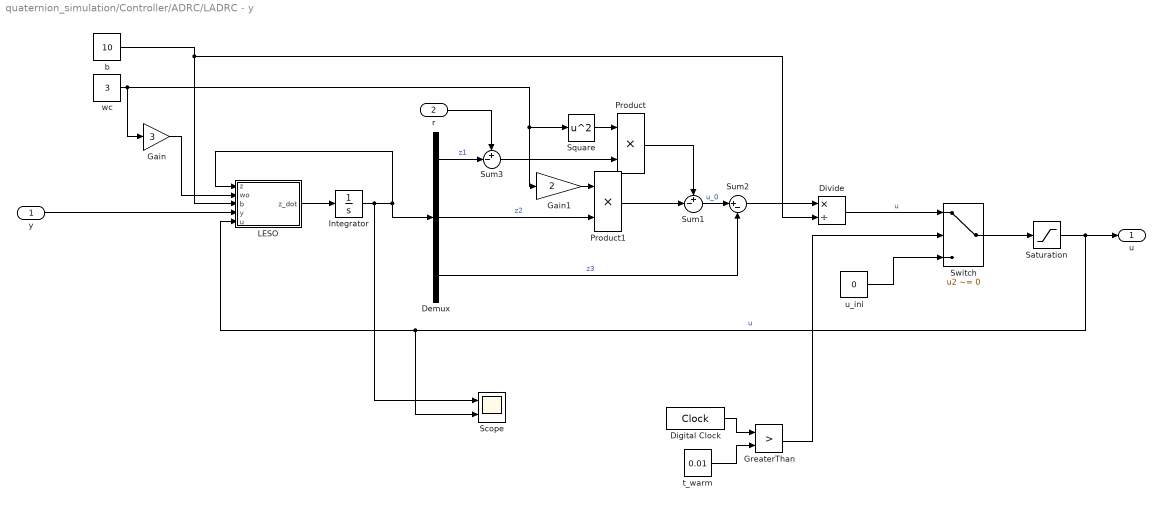
== system quaternion_simulation/Controller/ADRC/LADRC - y ==
  y : Inport
  r : Inport  Port=2
  Demux : Demux  Outputs=3
  Digital Clock : DigitalClock  SampleTime=Ts
  Divide : Product  Inputs=*/
  Gain : Gain  Gain=3
  Gain1 : Gain  Gain=2
  GreaterThan : RelationalOperator  Operator=>  OutDataTypeStr=boolean  RndMeth=Simplest  InputSameDT=off
  Integrator : Integrator  InitialCondition=[0 0 0]'
  LESO : MATLAB Function  TreatAsAtomicUnit=on
  Product : Product
  Product1 : Product
  Saturation : Saturate  UpperLimit=3  LowerLimit=-3
  Scope : Scope  NumInputPorts=2
  Square : Math  Operator=square
  Sum1 : Sum  Inputs=+-|
  Sum2 : Sum  Inputs=|+-
  Sum3 : Sum  Inputs=+-|
  Switch : Switch  Criteria=u2 ~= 0  Threshold=0.1  SaturateOnIntegerOverflow=off  InputSameDT=off
  b : Constant  Value=10
  t_warm : Constant  Value=0.01
  u_ini : Constant  Value=0  OutDataTypeStr=single
  wc : Constant  Value=3
  u : Outport
  wires:
  LESO/1(z_dot) -> Integrator/1
  Demux/1 -> Sum3/2  "z1"
  Product/1 -> Sum1/1
  Sum1/1 -> Sum2/1  "u_0"
  Demux/3 -> Sum2/2  "z3"
  Sum2/1 -> Divide/1
  Square/1 -> Product/1
  Gain1/1 -> Product1/1
  Demux/2 -> Product1/2  "z2"
  Product1/1 -> Sum1/2
  Saturation/1 -> Scope/2, LESO/5(u), u/1  "u"
  Switch/1 -> Saturation/1
  Divide/1 -> Switch/1  "u"
  u_ini/1 -> Switch/3
  r/1 -> Sum3/1
  Sum3/1 -> Product/2
  b/1 -> Divide/2, LESO/3(b)
  wc/1 -> Gain/1, Gain1/1, Square/1
  Gain/1 -> LESO/2(wo)
  t_warm/1 -> GreaterThan/2
  Digital Clock/1 -> GreaterThan/1
  GreaterThan/1 -> Switch/2
  y/1 -> LESO/4(y)
  Integrator/1 -> Scope/1, LESO/1(z), Demux/1

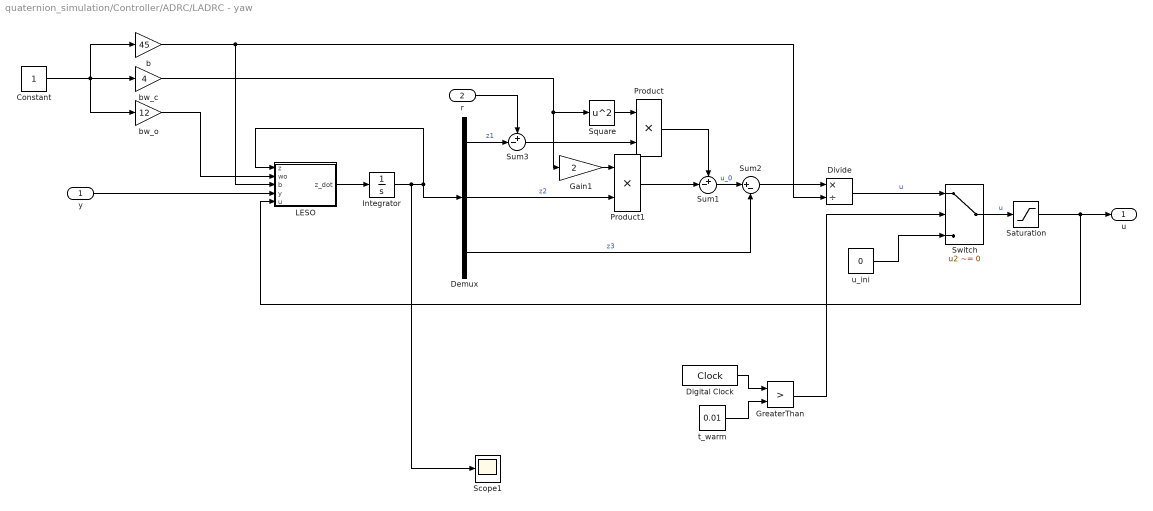
== system quaternion_simulation/Controller/ADRC/LADRC - yaw ==
  y : Inport
  r : Inport  Port=2
  Constant : Constant
  Demux : Demux  Outputs=3
  Digital Clock : DigitalClock  SampleTime=Ts
  Divide : Product  Inputs=*/
  Gain1 : Gain  Gain=2
  GreaterThan : RelationalOperator  Operator=>  OutDataTypeStr=boolean  RndMeth=Simplest  InputSameDT=off
  Integrator : Integrator  InitialCondition=[0 0 0]'
  LESO : MATLAB Function  TreatAsAtomicUnit=on
  Product : Product
  Product1 : Product
  Saturation : Saturate  UpperLimit=0.25  LowerLimit=-0.25
  Scope1 : Scope
  Square : Math  Operator=square
  Sum1 : Sum  Inputs=+-|
  Sum2 : Sum  Inputs=|+-
  Sum3 : Sum  Inputs=+-|
  Switch : Switch  Criteria=u2 ~= 0  Threshold=0.1  SaturateOnIntegerOverflow=off  InputSameDT=off
  b : Gain  Gain=45
  bw_c : Gain  Gain=4
  bw_o : Gain  Gain=12
  t_warm : Constant  Value=0.01
  u_ini : Constant  Value=0  OutDataTypeStr=single
  u : Outport
  wires:
  LESO/1(z_dot) -> Integrator/1
  Integrator/1 -> Scope1/1, LESO/1(z), Demux/1
  Demux/1 -> Sum3/2  "z1"
  Product/1 -> Sum1/1
  Sum1/1 -> Sum2/1  "u_0"
  Demux/3 -> Sum2/2  "z3"
  Sum2/1 -> Divide/1
  Square/1 -> Product/1
  Gain1/1 -> Product1/1
  Demux/2 -> Product1/2  "z2"
  Product1/1 -> Sum1/2
  Switch/1 -> Saturation/1  "u"
  Divide/1 -> Switch/1  "u"
  u_ini/1 -> Switch/3
  r/1 -> Sum3/1
  Sum3/1 -> Product/2
  b/1 -> Divide/2, LESO/3(b)
  bw_c/1 -> Gain1/1, Square/1
  bw_o/1 -> LESO/2(wo)
  t_warm/1 -> GreaterThan/2
  Digital Clock/1 -> GreaterThan/1
  GreaterThan/1 -> Switch/2
  y/1 -> LESO/4(y)
  Constant/1 -> bw_c/1, bw_o/1, b/1
  Saturation/1 -> LESO/5(u), u/1

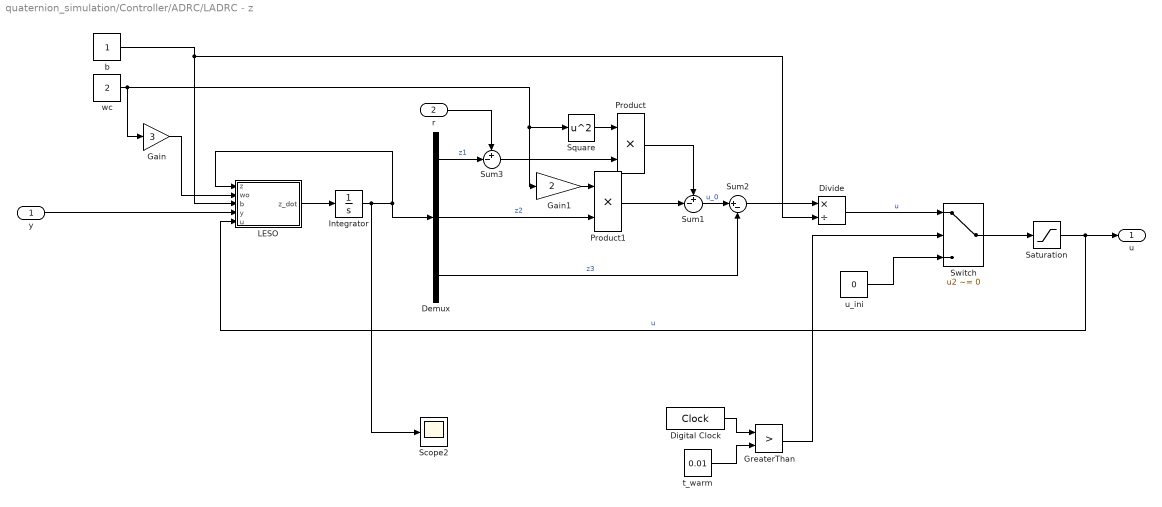
== system quaternion_simulation/Controller/ADRC/LADRC - z ==
  y : Inport
  r : Inport  Port=2
  Demux : Demux  Outputs=3
  Digital Clock : DigitalClock  SampleTime=Ts
  Divide : Product  Inputs=*/
  Gain : Gain  Gain=3
  Gain1 : Gain  Gain=2
  GreaterThan : RelationalOperator  Operator=>  OutDataTypeStr=boolean  RndMeth=Simplest  InputSameDT=off
  Integrator : Integrator  InitialCondition=[0 0 0]'
  LESO : MATLAB Function  TreatAsAtomicUnit=on
  Product : Product
  Product1 : Product
  Saturation : Saturate  UpperLimit=3  LowerLimit=-3
  Scope2 : Scope
  Square : Math  Operator=square
  Sum1 : Sum  Inputs=+-|
  Sum2 : Sum  Inputs=|+-
  Sum3 : Sum  Inputs=+-|
  Switch : Switch  Criteria=u2 ~= 0  Threshold=0.1  SaturateOnIntegerOverflow=off  InputSameDT=off
  b : Constant
  t_warm : Constant  Value=0.01
  u_ini : Constant  Value=0  OutDataTypeStr=single
  wc : Constant  Value=2
  u : Outport
  wires:
  LESO/1(z_dot) -> Integrator/1
  Integrator/1 -> Scope2/1, LESO/1(z), Demux/1
  Demux/1 -> Sum3/2  "z1"
  Product/1 -> Sum1/1
  Sum1/1 -> Sum2/1  "u_0"
  Demux/3 -> Sum2/2  "z3"
  Sum2/1 -> Divide/1
  Square/1 -> Product/1
  Gain1/1 -> Product1/1
  Demux/2 -> Product1/2  "z2"
  Product1/1 -> Sum1/2
  Saturation/1 -> LESO/5(u), u/1  "u"
  Switch/1 -> Saturation/1
  Divide/1 -> Switch/1  "u"
  u_ini/1 -> Switch/3
  r/1 -> Sum3/1
  Sum3/1 -> Product/2
  b/1 -> Divide/2, LESO/3(b)
  wc/1 -> Gain/1, Gain1/1, Square/1
  Gain/1 -> LESO/2(wo)
  t_warm/1 -> GreaterThan/2
  Digital Clock/1 -> GreaterThan/1
  GreaterThan/1 -> Switch/2
  y/1 -> LESO/4(y)

== matlab function quaternion_simulation/Controller/ADRC/LADRC - y/LESO ==
  data: z input; wo input; b input; z_dot output; y input; u input
function z_dot = LESO(z, wo, b, y, u)
    A = [0 1 0; 0 0 1; 0 0 0];
    B = [0 b 0]';
    C = [1 0 0];
    L = [3*wo 3*wo^2 wo^3]';
        
    z_dot = (A*z + B*u + L*(y-C*z));

== matlab function quaternion_simulation/Guidance/Trajectory Generator ==
  data: t input; x_d output
function x_d = fcn(t)

% if t < 5
%     temp = [1 2 0 0 0 0];
% elseif 20 <= t
%     temp = [1 2 0 0 0 0];
% elseif 15 <= t
%     temp = [1 3 0 0 0 0];
% elseif 10 <= t
%     temp = [2 3 1 0 0 0];
% elseif 5 <= t
%     temp = [2 2 0 0 0 0];
% else
%     temp = [90 90 90 0 0 0];
% end
% x = sin(t);
% y = cos(t);
if t < 1.5
    temp = [0 0 0 0 0 0];
elseif 10 >= t
    temp = [0 0 1.5 0 0 0];
elseif 20 >= t
    temp = [0 -1 1.5 0 0 0];
elseif 30 >= t
    temp = [-1 -1 1.5 0 0 0];
elseif 40 >= t
    temp = [-1 0 1.5 0 0 0];
elseif 50 >= t
    temp = [0 0 1.5 0 0 0];
elseif 60 >= t
    landing = 1.5 - 1.5*(t-50)/10;
    temp = [0 0 landing 0 0 0];
else
    temp = [0 0 0 0 0 0];
end
% temp = [1+x 2+y 0 0 0 0];
x_d = temp;

== matlab function quaternion_simulation/Controller/ADRC/LADRC - dX/LESO ==
  data: z input; wo input; b input; z_dot output; y input; u input
function z_dot = LESO(z, wo, b, y, u)
    A = [0 1 0; 0 0 1; 0 0 0];
    B = [0 b 0]';
    C = [1 0 0];
    L = [3*wo 3*wo^2 wo^3]';
        
    z_dot = (A*z + B*u + L*(y-C*z));

== matlab function quaternion_simulation/Controller/State-Feedback/Quaternion to Axis Angle ==
  data: q input; theta output
function theta = fcn(q)
    temp = [0 0 0]';
    
    if norm(q(2:4))
        temp = q(2:4)/norm(q(2:4))*acos(q(1));
    end
    
theta = 2 * temp;

== matlab function quaternion_simulation/Controller/ADRC/LADRC - z/LESO ==
  data: z input; wo input; b input; z_dot output; y input; u input
function z_dot = LESO(z, wo, b, y, u)
    A = [0 1 0; 0 0 1; 0 0 0];
    B = [0 b 0]';
    C = [1 0 0];
    L = [3*wo 3*wo^2 wo^3]';
        
    z_dot = (A*z + B*u + L*(y-C*z));

== matlab function quaternion_simulation/Controller/ADRC/LADRC - x/LESO ==
  data: z input; wo input; b input; z_dot output; y input; u input
function z_dot = LESO(z, wo, b, y, u)
    A = [0 1 0; 0 0 1; 0 0 0];
    B = [0 b 0]';
    C = [1 0 0];
    L = [3*wo 3*wo^2 wo^3]';
        
    z_dot = (A*z + B*u + L*(y-C*z));

== matlab function quaternion_simulation/Controller/ADRC/LADRC - dY/LESO ==
  data: z input; wo input; b input; z_dot output; y input; u input
function z_dot = LESO(z, wo, b, y, u)
    A = [0 1 0; 0 0 1; 0 0 0];
    B = [0 b 0]';
    C = [1 0 0];
    L = [3*wo 3*wo^2 wo^3]';
        
    z_dot = (A*z + B*u + L*(y-C*z));

== matlab function quaternion_simulation/Controller/ADRC/LADRC - yaw/LESO ==
  data: z input; wo input; b input; z_dot output; y input; u input
function z_dot = LESO(z, wo, b, y, u)
    A = [0 1 0; 0 0 1; 0 0 0];
    B = [0 b 0]';
    C = [1 0 0];
    L = [3*wo 3*wo^2 wo^3]';
        
    z_dot = (A*z + B*u + L*(y-C*z));

== matlab function quaternion_simulation/Plant/Model ==
  data: x input; u input; x_dot output; m input; J input; disturbance input
function x_dot = dynamics(x, u, m, J, disturbance)
% x = transpose(x);
% x = [X, Y, Z, dX, dY, dZ, q0, q1, q2, q3, wX, wY, wZ]
% u = [F_th, tX, tY, Tz]

q = quaternion(x(7:10)');
q_omega = quaternion([0 x(11:13)']);
q_thrust = quaternion([0 0 0 u(1)]/m);

lin_vel = x(4:6);
lin_acc = compact(q*q_thrust*q.conj);
lin_acc = lin_acc(2:4) + [0 0 -9.81] + disturbance;
ang_vel = compact(0.5 * q * q_omega);
ang_acc = inv(J)*(u(2:4) - cross(x(11:13), J*x(11:13)));

x_dot = [lin_vel; lin_acc'; ang_vel'; ang_acc];

== matlab function quaternion_simulation/Controller/State-Feedback/Control Input to Torque ==
  data: J input; u input; omega input; tau output
function tau = fcn(J, u, omega)
    % tau = J*u + omega x J*omega
    temp = J * u + cross(omega, J*omega);
tau = temp;

== matlab function quaternion_simulation/Controller/State-Feedback/u_pd to F_th ==
  data: m input; F_th output; u_pd input
function F_th = fcn(m, u_pd)
    b = [0 0 1]';
    temp = b * norm(u_pd) * m;
F_th = temp(3);

== matlab function quaternion_simulation/Plant/MATLAB Function1 ==
  data: q0_in input; q0 output; q1_in input; q2_in input; q3_in input; q1 output; q2 output; q3 output
function [q0, q1, q2, q3] = fcn(q0_in, q1_in, q2_in, q3_in)
    d = norm([q0_in q1_in q2_in q3_in]);
    
 q0 = q0_in / d;
 q1 = q1_in / d;
 q2 = q2_in / d;
 q3 = q3_in / d;
% [q0, q1, q2, q3] = [q0_in q1_in q2_in q3_in]/d;

== matlab function quaternion_simulation/Controller/State-Feedback/Desired Position to Desired Angle ==
  data: up input; theta output
function theta = fcn(up)
    
    
    b = [0 0 1];
    q_d = quaternion([(b * up + norm(up)) cross(b, up)]);
    
    q = compact(q_d.normalize);
    theta = [0 0 0];
       
    % eq. (5) in J.Carino, et al.
    if norm(q(2:4))       
        ln_q = q(2:4)/norm(q(2:4))*acos(q(1));
        theta = 2 * ln_q;
    end

== matlab function quaternion_simulation/Controller/ADRC/LADRC - dZ/LESO ==
  data: z input; wo input; b input; z_dot output; y input; u input
function z_dot = LESO(z, wo, b, y, u)
    A = [0 1 0; 0 0 1; 0 0 0];
    B = [0 b 0]';
    C = [1 0 0];
    L = [3*wo 3*wo^2 wo^3]';
        
    z_dot = (A*z + B*u + L*(y-C*z));

== matlab function quaternion_simulation/Controller/ADRC/LADRC - roll/LESO ==
  data: z input; wo input; b input; z_dot output; y input; u input
function z_dot = LESO(z, wo, b, y, u)
    A = [0 1 0; 0 0 1; 0 0 0];
    B = [0 b 0]';
    C = [1 0 0];
    L = [3*wo 3*wo^2 wo^3]';
        
    z_dot = (A*z + B*u + L*(y-C*z));

== matlab function quaternion_simulation/Controller/ADRC/LADRC - pitch/LESO ==
  data: z input; wo input; b input; z_dot output; y input; u input
function z_dot = LESO(z, wo, b, y, u)
    A = [0 1 0; 0 0 1; 0 0 0];
    B = [0 b 0]';
    C = [1 0 0];
    L = [3*wo 3*wo^2 wo^3]';
        
    z_dot = (A*z + B*u + L*(y-C*z));
